simulink library "APN_Battery_Lib"  (R2014a)
settings: Solver=ode45  StartTime=0.0  StopTime=10.0  RelTol=1e-3
undefined symbols (not defined in the file): Emo, Kt, Kt_Temps, theta_f, theta_init
libraries: fl_lib x8, LeadAcidBattery_lib x6, nesl_utility x3
Description:
  | Copyright 2014 The MathWorks, Inc.
settings Model: Creator=smiller  LastModifiedBy=psanghvi

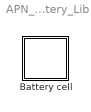
== system APN_Battery_Lib ==
  Battery cell : Subsystem
      mask Display:
      | image(imread('battery.jpg'))
      | color('red')
      | port_label('LConn',1,'+')
      | port_label('LConn',2,'H')
      | port_label('RConn',1,'-')

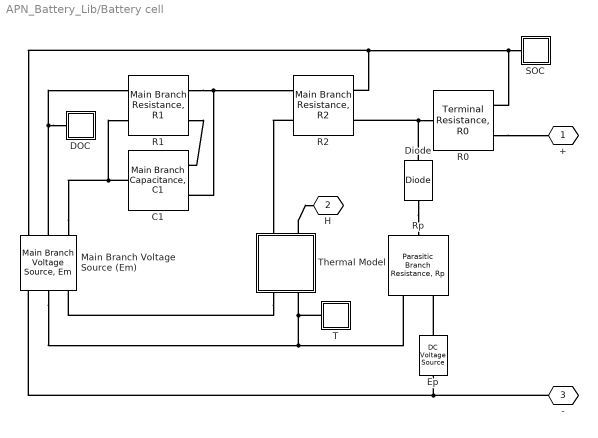
== system APN_Battery_Lib/Battery cell ==
  " DOC " : Subsystem
  " SOC " : Subsystem
  C1 : LeadAcidBattery_lib/Main Branch Capacitance, C1  Tau1=Tau1 s  Cmin=1e-5 F
  Diode : fl_lib/Electrical/Electrical Elements/Diode  Vf=0.6 V  Ron=0.3 Ohm  Goff=1e-08 1/Ohm  i_specify=off  i_priority=High  i=0 A  v_specify=off  v_priority=High  v=0 V
  Ep : fl_lib/Electrical/Electrical Sources/DC Voltage Source  v0=Ep V
  Main Branch Voltage Source (Em) : LeadAcidBattery_lib/Main Branch Voltage Source, Em  Em0=Emo*14 V  Ke=Ke V/K  Kc=Kc  C0=Costar s*A  Istar=Istar A  delta=delta  Tau1=Tau1 s  Qinit=Qe_init s*A
  R0 : LeadAcidBattery_lib/Terminal Resistance, R0  R00=Roo Ohm  A0=Ao
  R1 : LeadAcidBattery_lib/Main Branch Resistance, R1  R10=R10 Ohm  DOC_min=1e-006
  R2 : LeadAcidBattery_lib/Main Branch Resistance, R2  R20=R20 Ohm  A21=A21  A22=A22  Istar=Istar A
  Rp : LeadAcidBattery_lib/Parasitic Branch Resistance, Rp  Gp0=Gpo 1/Ohm  Vp0=Vpo V  Ap=Ap  Tf=theta_f C
  T : Subsystem
  Thermal Model : Subsystem
  + : PMIOPort  Tag=PMCPort  Port=1  Side=Left
  H : PMIOPort  Tag=PMCPort  Port=2  Side=Left
  - : PMIOPort  Tag=PMCPort  Port=3  Side=Right
  connections:
  Diode/LConn1 -- R0/RConn1 -- R2/LConn2
  R2/RConn2 -- Thermal Model/LConn1
  -/RConn1 -- Ep/RConn1 -- Main Branch Voltage Source (Em)/RConn1
  Thermal Model/RConn1 -- Main Branch Voltage Source (Em)/RConn3
  Diode/RConn1 -- Rp/LConn1
  Ep/LConn1 -- Rp/RConn2
  Thermal Model/LConn2 -- H/RConn1
  " SOC "/LConn1 -- R0/LConn1 -- R2/LConn1 -- Main Branch Voltage Source (Em)/LConn1
  R1/LConn2 -- C1/LConn1
  R1/LConn1 -- C1/LConn2 -- R2/RConn1
  Main Branch Voltage Source (Em)/LConn3 -- R1/RConn2 -- C1/RConn1
  " DOC "/LConn1 -- R1/RConn1 -- Main Branch Voltage Source (Em)/LConn2
  R0/LConn2 -- +/RConn1
  Main Branch Voltage Source (Em)/RConn2 -- Rp/RConn1 -- Thermal Model/RConn2 -- T/LConn1

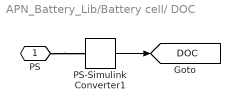
== system APN_Battery_Lib/Battery cell/ DOC  ==
  PS-Simulink Converter1 : nesl_utility/PS-Simulink Converter  PhysicalDomain=network_engine_domain  SubClassName=ps_output  LeftPortType=input  RightPortType=output  PseudoPeriodic=off  Frequencies=[]  Unit=1  AffineConversion=off
  PS : PMIOPort  Port=1  Side=Left
  tag scope: DOC=global
  wires:
  PS-Simulink Converter1/1 -> [DOC]
  connections:
  PS/RConn1 -- PS-Simulink Converter1/LConn1

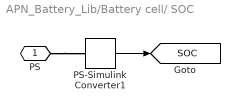
== system APN_Battery_Lib/Battery cell/ SOC  ==
  PS-Simulink Converter1 : nesl_utility/PS-Simulink Converter  PhysicalDomain=network_engine_domain  SubClassName=ps_output  LeftPortType=input  RightPortType=output  PseudoPeriodic=off  Frequencies=[]  Unit=1  AffineConversion=off
  PS : PMIOPort  Port=1  Side=Left
  tag scope: SOC=global
  wires:
  PS-Simulink Converter1/1 -> [SOC]
  connections:
  PS/RConn1 -- PS-Simulink Converter1/LConn1

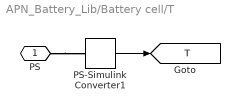
== system APN_Battery_Lib/Battery cell/T ==
  PS-Simulink Converter1 : nesl_utility/PS-Simulink Converter  PhysicalDomain=network_engine_domain  SubClassName=ps_output  LeftPortType=input  RightPortType=output  PseudoPeriodic=off  Frequencies=[]  Unit=C  AffineConversion=on
  PS : PMIOPort  Port=1  Side=Left
  tag scope: T=global
  wires:
  PS-Simulink Converter1/1 -> [T]
  connections:
  PS/RConn1 -- PS-Simulink Converter1/LConn1

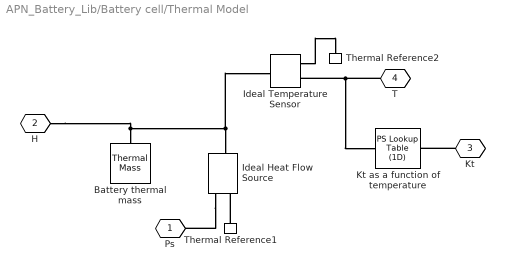
== system APN_Battery_Lib/Battery cell/Thermal Model ==
  Battery thermal mass : fl_lib/Thermal/Thermal Elements/Thermal Mass  mass=1 kg  sp_heat=Ctheta J/kg/K  Q_specify=off  Q_priority=High  Q=0 J/s  T_specify=on  T_priority=High  T=theta_init+273 K
  Ideal Temperature Sensor : fl_lib/Thermal/Thermal Sensors/Ideal Temperature Sensor
  Ideal Heat Flow Source : fl_lib/Thermal/Thermal Sources/Ideal Heat Flow Source
  Kt as a function of temperature : fl_lib/Physical Signals/Lookup Tables/PS Lookup Table (1D)  x_t=[theta_f, Kt_Temps]+273  y_t=[0 Kt]  interp_method=1  extrap_method=1
  Thermal Reference1 : fl_lib/Thermal/Thermal Elements/Thermal Reference
  Thermal Reference2 : fl_lib/Thermal/Thermal Elements/Thermal Reference
  Ps : PMIOPort  Tag=PMCPort  Port=1  Side=Left
  H : PMIOPort  Tag=PMCPort  Port=2  Side=Left
  Kt : PMIOPort  Tag=PMCPort  Port=3  Side=Right
  T : PMIOPort  Tag=PMCPort  Port=4  Side=Right
  connections:
  Ideal Heat Flow Source/RConn1 -- Ps/RConn1
  Kt/RConn1 -- Kt as a function of temperature/RConn1
  Battery thermal mass/LConn1 -- Ideal Heat Flow Source/LConn1 -- Ideal Temperature Sensor/LConn1 -- H/RConn1
  Thermal Reference1/LConn1 -- Ideal Heat Flow Source/RConn2
  T/RConn1 -- Kt as a function of temperature/LConn1 -- Ideal Temperature Sensor/RConn2
  Ideal Temperature Sensor/RConn1 -- Thermal Reference2/LConn1
